simulink model "motor_velocity_interface"  (R2019b)
settings: Solver=FixedStepAuto  StartTime=0.0  StopTime=25  FixedStep=FIXED_STEP_SIZE  RelTol=1e-3
model workspace (MAT data in the model file):
  SL_ROS_VariableLengthArrays_MaxSizes.CommonInfo.ArrayTruncateAction = 'EmitWarning'
  SL_ROS_VariableLengthArrays_MaxSizes.MsgTypeMap = containers.Map
  SL_ROS_VariableLengthArrays_MaxSizes.MsgTypeMap.serialization.keys = {'mav_msgs/Actuators'}
  SL_ROS_VariableLengthArrays_MaxSizes.MsgTypeMap.serialization.values{1}(1).PropertyName = 'Angles'
  SL_ROS_VariableLengthArrays_MaxSizes.MsgTypeMap.serialization.values{1}(1).DataType = 'double'
  SL_ROS_VariableLengthArrays_MaxSizes.MsgTypeMap.serialization.values{1}(1).MaxLength = 128
  SL_ROS_VariableLengthArrays_MaxSizes.MsgTypeMap.serialization.values{1}(2).PropertyName = 'AngularVelocities'
  SL_ROS_VariableLengthArrays_MaxSizes.MsgTypeMap.serialization.values{1}(2).DataType = 'double'
  SL_ROS_VariableLengthArrays_MaxSizes.MsgTypeMap.serialization.values{1}(2).MaxLength = 4
  SL_ROS_VariableLengthArrays_MaxSizes.MsgTypeMap.serialization.values{1}(3).PropertyName = 'Normalized'
  SL_ROS_VariableLengthArrays_MaxSizes.MsgTypeMap.serialization.values{1}(3).DataType = 'double'
  SL_ROS_VariableLengthArrays_MaxSizes.MsgTypeMap.serialization.values{1}(3).MaxLength = 128
  SL_ROS_VariableLengthArrays_MaxSizes.MsgTypeMap.serialization.uniformity = 0
  SL_ROS_VariableLengthArrays_MaxSizes.MsgTypeMap.serialization.keyType = 'char'
  SL_ROS_VariableLengthArrays_MaxSizes.MsgTypeMap.serialization.valueType = 'any'
values from neighbouring files (symbols this model uses):
  attMtx = [L*k, 0, -L*k, 0; 0, L*k, 0, -L*k; b, -b, b, -b; 1, 1, 1, 1]    [Ex6_5.m]
  FIXED_STEP_SIZE = 0.01    [Ex6_5.m]
  g = 9.81    [Ex6_5.m]
  k = 8.54858e-06    [Ex6_5.m]
  m = 0.716    [Ex6_5.m]
undefined symbols (not defined in the file or in its folder): AngularVelocities, AngularVelocities_SL_Info, Header
libraries: robotlib x5, robotgazebolib x1, simulink x1
settings Model: Creator=ananda  LastModifiedBy=harsh
settings OptimizationCC: EnhancedBackFolding=on  PassReuseOutputArgsAs=Individual arguments  ZeroExternalMemoryAtStartup=off  ZeroInternalMemoryAtStartup=off  MaxStackSize=64  OptimizeBlockOrder=speed  DifferentSizesBufferReuse=on  OptimizationCustomize=off  EfficientTunableParamExpr=on
settings DebuggingCC: ParameterTunabilityLossMsg=error
settings HardwareCC: ProdBitPerPointer=32  ProdBitPerSizeT=32  ProdBitPerPtrDiffT=32  ProdLargestAtomicFloat=None  ProdIntDivRoundTo=Undefined  ProdEndianess=Unspecified  ProdWordSize=32  ProdHWDeviceType=Generic->Unspecified (assume 32-bit Generic)  UseEmbeddedCoderFeatures=off
settings SFSimCC: MATLABDynamicMemAlloc=off
settings RTWCC: SystemTargetFile=ert.tlc  HardwareBoard=Robot Operating System (ROS)  TLCOptions="-aInlineSetEventsForThisBaseRateFcn=TLC_FALSE -aSuppressMultiTaskScheduler=TLC_FALSE  -aRateBasedStepFcn=0"  TemplateMakefile=ert_default_tmf  GenerateReport=on  Toolchain=Catkin  IncludeHyperlinkInReport=on  LaunchReport=on  TargetLang=C++  GenerateTraceInfo=on  GenerateTraceReport=on  GenerateTraceReportSl=on  GenerateTraceReportSf=on  GenerateTraceReportEml=on
settings CodeAppCC: ForceParamTrailComments=on  IgnoreCustomStorageClasses=off  OperatorAnnotations=on  SimulinkDataObjDesc=on  SFDataObjDesc=on  InsertBlockDesc=on
settings ERTTargetCC: SupportNonInlinedSFcns=on

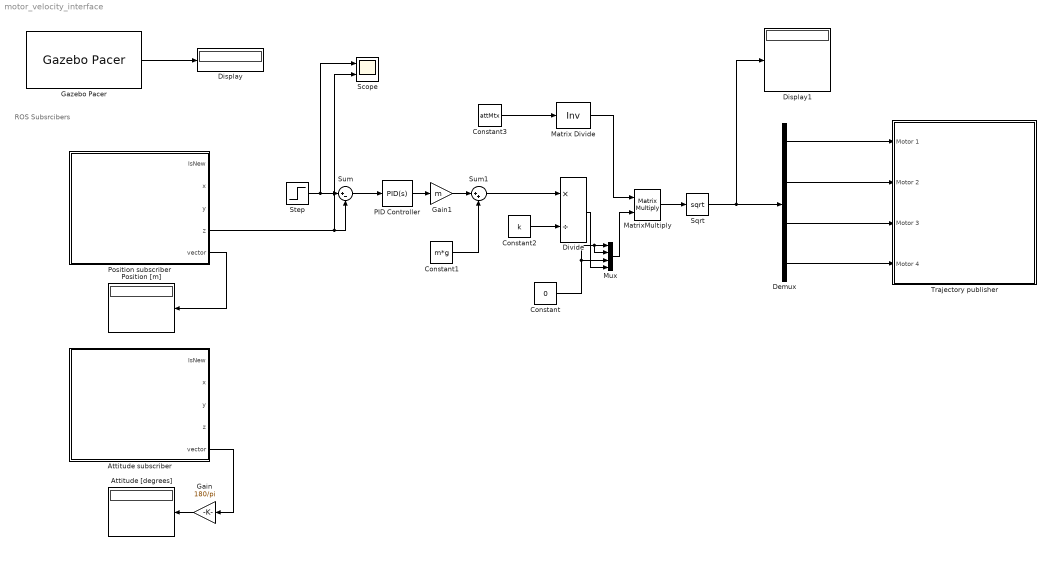
== system motor_velocity_interface ==
  note: ROS Subsrcibers
  Attitude [degrees] : Display
  Attitude subscriber : Subsystem
  Constant : Constant  Value=0
  Constant1 : Constant  Value=m*g
  Constant2 : Constant  Value=k
  Constant3 : Constant  Value=attMtx
  Demux : Demux
  Display : Display
  Display1 : Display
  Divide : Product  Inputs=*/
  Gain : Gain  Gain=180/pi
  Gain1 : Gain  Gain=m
  Gazebo Pacer : robotgazebolib/Gazebo Pacer  ResetBehavior=Reset Gazebo simulation time  SampleTime=FIXED_STEP_SIZE
      settings: SourceProductName=Robotics System Toolbox  SourceProductBaseCode=RO
  Matrix Divide : Product  Inputs=/  Multiplication=Matrix(*)
  MatrixMultiply : Product  Multiplication=Matrix(*)
  Mux : Mux
  PID Controller : simulink/Continuous/PID Controller  Controller=PID  Form=Parallel  TimeDomain=Continuous-time  SampleTime=-1  IntegratorMethod=Forward Euler  FilterMethod=Forward Euler  ControllerParametersSource=internal  P=5  I=0.5  D=2  UseFilter=on  N=100  TunerSelectOption=Transfer Function Based (PID Tuner App)  InitialConditionSource=internal  InitialConditionForIntegrator=0  InitialConditionForFilter=0  DifferentiatorICPrevScaledInput=0  ExternalReset=none  TrackingMode=off  Kt=1  LimitOutput=off  UpperSaturationLimit=inf  LowerSaturationLimit=-inf  LinearizeAsGain=on  AntiWindupMode=none  Kb=1  POutMin=[]  POutMax=[]  IOutMin=[]  IOutMax=[]  DOutMin=[]  DOutMax=[]  NOutMin=[]  NOutMax=[]  SumOutMin=[]  SumOutMax=[]  SaturationOutMin=[]  SaturationOutMax=[]  PParamMin=[]  PParamMax=[]  IParamMin=[]  IParamMax=[]  DParamMin=[]  DParamMax=[]  NParamMin=[]  NParamMax=[]  KbParamMin=[]  KbParamMax=[]  KtParamMin=[]  KtParamMax=[]  KbOutMin=[]  KbOutMax=[]  KtOutMin=[]  KtOutMax=[]  IntegratorOutMin=[]  IntegratorOutMax=[]  FilterOutMin=[]  FilterOutMax=[]  SumI1OutMin=[]  SumI1OutMax=[]  SumI2OutMin=[]  SumI2OutMax=[]  SumI3OutMin=[]  SumI3OutMax=[]  SumI4OutMin=[]  SumI4OutMax=[]  SumDOutMin=[]  SumDOutMax=[]  DifferentiatorOutMin=[]  DifferentiatorOutMax=[]  FilterDiffOutCoefMin=[]  FilterDiffOutCoefMax=[]  ReciprocalOutMin=[]  ReciprocalOutMax=[]  SumDenOutMin=[]  SumDenOutMax=[]  SumNumOutMin=[]  SumNumOutMax=[]  DivideOutMin=[]  DivideOutMax=[]  IntegratorContinuousStateAttributes=''  IntegratorStateMustResolveToSignalObject=off  IntegratorRTWStateStorageClass=Auto  FilterContinuousStateAttributes=''  FilterStateMustResolveToSignalObject=off  FilterRTWStateStorageClass=Auto  ParallelPVariant=InternalParameters  IdealPVariant=Disabled  IVariant=InternalParameters  DVariant=InternalParameters  IntegratorVariant=Continuous  SatVariant=Disabled  AWVariant=Passthrough  PCopyVariant=Disabled  TRVariant=Disabled  FdbkBlocksVariant=Forward  IdealPFdbkVariant=Disabled  SatFdbkVariant=Disabled  DerivativeFilterVariant=ContFilter  NVariant=InternalParameters  NCopyVariant=Disabled  FilterICVariant=InternalICsFilter  IntegratorICVariant=InternalICs  ExternalResetVariant=Disabled  TRSumVariant=Passthrough  SumFdbkVariant=Disabled  SumVariant=Sum_PID
  Position [m] : Display
  Position subscriber : Subsystem
  Scope : Scope  NumInputPorts=2
  Sqrt : Sqrt  SaturateOnIntegerOverflow=on
  Step : Step  SampleTime=0
  Sum : Sum  Inputs=|+-
  Sum1 : Sum  Inputs=|++
  Trajectory publisher : Subsystem
  wires:
  Position subscriber/5(vector) -> Position [m]/1
  Attitude subscriber/5(vector) -> Gain/1
  Gain/1 -> Attitude [degrees]/1
  Gazebo Pacer/1 -> Display/1
  Position subscriber/4(z) -> Scope/2, Sum/2
  Step/1 -> Scope/1, Sum/1
  Sum/1 -> PID Controller/1
  PID Controller/1 -> Gain1/1
  Gain1/1 -> Sum1/1
  Constant1/1 -> Sum1/2
  Sum1/1 -> Divide/1
  Constant2/1 -> Divide/2
  Constant3/1 -> Matrix Divide/1
  Matrix Divide/1 -> MatrixMultiply/1
  Divide/1 -> Mux/4
  MatrixMultiply/1 -> Sqrt/1
  Demux/1 -> Trajectory publisher/1(Motor 1)
  Demux/2 -> Trajectory publisher/2(Motor 2)
  Demux/3 -> Trajectory publisher/3(Motor 3)
  Demux/4 -> Trajectory publisher/4(Motor 4)
  Sqrt/1 -> Demux/1, Display1/1
  Constant/1 -> Mux/1, Mux/2, Mux/3
  Mux/1 -> MatrixMultiply/2

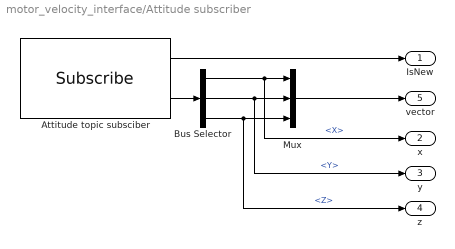
== system motor_velocity_interface/Attitude subscriber ==
  Attitude topic subsciber : robotlib/Subscribe  topicSource=Specify your own  topic=/hummingbird/orientation_rpy  messageType=geometry_msgs/Vector3  sampleTime=ATTI_SUB_DT  messageQueueLength=1
      settings: SourceProductName=ROS Toolbox
  Bus Selector : BusSelector  OutputSignals=X,Y,Z
  Mux : Mux  Inputs=3
  IsNew : Outport
  x : Outport  Port=2
  y : Outport  Port=3
  z : Outport  Port=4
  vector : Outport  Port=5
  wires:
  Bus Selector/3 -> z/1, Mux/3  "<Z>"
  Bus Selector/2 -> y/1, Mux/2  "<Y>"
  Bus Selector/1 -> x/1, Mux/1  "<X>"
  Attitude topic subsciber/2 -> Bus Selector/1
  Attitude topic subsciber/1 -> IsNew/1
  Mux/1 -> vector/1

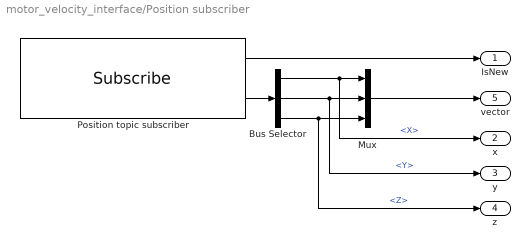
== system motor_velocity_interface/Position subscriber ==
  Bus Selector : BusSelector  OutputSignals=Point.X,Point.Y,Point.Z
  Mux : Mux  Inputs=3
  Position topic subscriber : robotlib/Subscribe  topicSource=Specify your own  topic=/hummingbird/odometry_sensor1/position  messageType=geometry_msgs/PointStamped  sampleTime=POS_SUB_DT  messageQueueLength=1
      settings: SourceProductName=ROS Toolbox
  IsNew : Outport
  x : Outport  Port=2
  y : Outport  Port=3
  z : Outport  Port=4
  vector : Outport  Port=5
  wires:
  Bus Selector/3 -> z/1, Mux/3  "<Z>"
  Bus Selector/2 -> y/1, Mux/2  "<Y>"
  Mux/1 -> vector/1
  Bus Selector/1 -> x/1, Mux/1  "<X>"
  Position topic subscriber/2 -> Bus Selector/1
  Position topic subscriber/1 -> IsNew/1

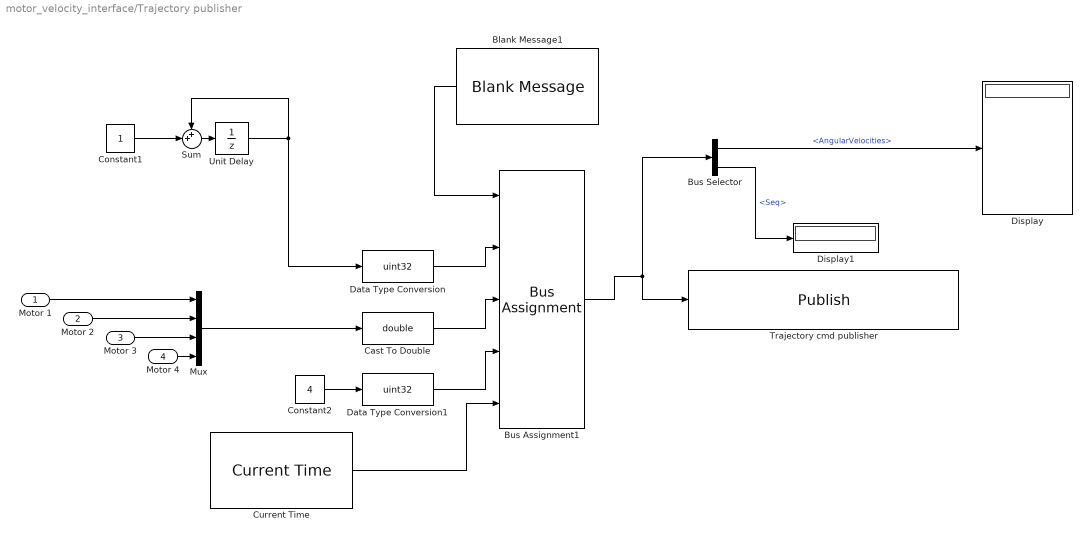
== system motor_velocity_interface/Trajectory publisher ==
  Motor 1 : Inport
  Motor 2 : Inport  Port=2
  Motor 3 : Inport  Port=3
  Motor 4 : Inport  Port=4
  Blank Message1 : robotlib/Blank Message  messageClass=Message  entityType=mav_msgs/Actuators  messageType=mav_msgs/Actuators  SampleTime=inf
      settings: SourceProductName=ROS Toolbox
  Bus Assignment1 : BusAssignment  AssignedSignals=Header.Seq,AngularVelocities,AngularVelocities_SL_Info.CurrentLength,Header.Stamp
  Bus Selector : BusSelector  OutputSignals=AngularVelocities,Header.Seq
  Cast To Double : DataTypeConversion  OutDataTypeStr=double
  Constant1 : Constant
  Constant2 : Constant  Value=4
  Current Time : robotlib/Current Time  OutputFormat=bus  SampleTime=FIXED_STEP_SIZE  ModelName=motor_velocity_interface
      settings: SourceProductName=ROS Toolbox  SourceProductBaseCode=RR
  Data Type Conversion : DataTypeConversion  OutDataTypeStr=uint32
  Data Type Conversion1 : DataTypeConversion  OutDataTypeStr=uint32
  Display : Display
  Display1 : Display
  Mux : Mux
  Sum : Sum  Inputs=++|
  Trajectory cmd publisher : robotlib/Publish  topicSource=Specify your own  topic=/hummingbird/command/motor_speed  messageType=mav_msgs/Actuators  messageQueueLength=1
      settings: SourceProductName=ROS Toolbox
  Unit Delay : UnitDelay  SampleTime=FIXED_STEP_SIZE  HasFrameUpgradeWarning=on
  wires:
  Bus Assignment1/1 -> Trajectory cmd publisher/1, Bus Selector/1
  Blank Message1/1 -> Bus Assignment1/1
  Data Type Conversion/1 -> Bus Assignment1/2
  Mux/1 -> Cast To Double/1
  Cast To Double/1 -> Bus Assignment1/3
  Bus Selector/1 -> Display/1  "<AngularVelocities>"
  Bus Selector/2 -> Display1/1  "<Seq>"
  Constant2/1 -> Data Type Conversion1/1
  Data Type Conversion1/1 -> Bus Assignment1/4
  Motor 1/1 -> Mux/1
  Motor 2/1 -> Mux/2
  Motor 3/1 -> Mux/3
  Motor 4/1 -> Mux/4
  Current Time/1 -> Bus Assignment1/5
  Sum/1 -> Unit Delay/1
  Unit Delay/1 -> Data Type Conversion/1, Sum/1
  Constant1/1 -> Sum/2
